simulink model "testEmplanner_cs"  (R2021b)
settings: Solver=ode5  StartTime=0.0  StopTime=60  FixedStep=1/1000  RelTol=1e-3
PreLoadFcn:
  | mbxruntime.callbacks.PreLoadFcn(bdroot);
PostLoadFcn:
  | mbxruntime.callbacks.PostLoadFcn(bdroot);
InitFcn:
  | mbxruntime.callbacks.InitFcn(bdroot);
StartFcn:
  | mbxruntime.callbacks.StartFcn(bdroot);
StopFcn:
  | mbxruntime.callbacks.StopFcn(bdroot);
model workspace (MAT data in the model file):
  mbox_table : object (value not decoded)
  model_closed = 0
  sim_status = 0
values from neighbouring files (symbols this model uses):
  c_factor = 43.75    [emplanner_init.m]
  cf = -175016    [emplanner_init.m]
  cr = -130634    [emplanner_init.m]
  global_path_x = [-1.1448 -0.145417744933 0.852705365581 1.84955224935 2.84511712279 3.83939835808 4.83239585569 5.82411007764 6.81454169183 7.80369144113 8.79156009523 9.77814843293 ... (3001 elements, 3001x1)]    [global_path.mat]
  global_path_y = [14.6488 14.6488 14.6488 14.6488 14.6488 14.6488 14.6488 14.6488 14.6488 14.6488 14.6488 14.6488 ... (3001 elements, 3001x1)]    [global_path.mat]
  KD_PID_distance = 0.0    (= 0)    [emplanner_init.m]
  KD_PID_speed = 0    [emplanner_init.m]
  KI_PID_distance = 0.0    (= 0)    [emplanner_init.m]
  KI_PID_speed = 0    [emplanner_init.m]
  KP_PID_distance = 0.5    [emplanner_init.m]
  KP_PID_speed = 1.8    [emplanner_init.m]
  la = 1.265    [emplanner_init.m]
  lb = 2.947-1.265    (= 1.682)    [emplanner_init.m]
  LQR_K1 = k(:,1)'    [emplanner_init.m]
  LQR_K2 = k(:,2)'    [emplanner_init.m]
  LQR_K3 = k(:,3)'    [emplanner_init.m]
  LQR_K4 = k(:,4)'    [emplanner_init.m]
  m = 2020    [emplanner_init.m]
  rack_displacement = [-39.14 , -37.2 , -35.29 , -33.43 , -31.6 , -29.81 , -28.06 , -26.34 , -24.66 ,      -23.01 , -21.38 , -19.79 , -18.23 , -16.69 , -15.18 , -13.7 , -12.23 , -10.8 , -9.38 , -7.98 ,     -6.61 , -5.25 , -3.91 , -2.59 , -1.29 , 0 , 1.27 , 2.54 , 3.78 , 5.02 , 6.24 , 7.46 , 8.66 ,      9.86 , 11.05 , 12.24 , 13.41 , 14.59 , 15.76 , 16.92 , 18.09 , 19.25 , 20.42 , 21.59 , 22.76 ,      23.93 , 25.11 , 26 ...(+26 chars)    [emplanner_init.m]
  right_wheel_ground = [-70 ,-67.2 , -64.4 , -61.6 , -58.8 , -56 , -53.2 , -50.4 , -47.6 , -44.8 , -42 ,      -39.2 , -36.4 , -33.6 , -30.8 , -28 , -25.2 , -22.4 , -19.6 , -16.8 , -14 , -11.2 , -8.4 , -5.6 ,      -2.8 , 0 , 2.8 , 5.6 , 8.4 , 11.2 , 14 , 16.8 , 19.6 , 22.4 , 25.2 , 28 , 30.8 , 33.6 , 36.4 ,      39.2 , 42 , 44.8 , 47.6 , 50.4 , 53.2 , 56 , 58.8 , 61.6 , 64.4 , 67.2 , 70 ]    [emplanner_init.m]
  vx_break_point = zeros(1,5000)    [emplanner_init.m]
undefined symbols (not defined in the file or in its folder): aubr, DiscIntNeverNeededParam, tablebr, vubr, warningInitialVelocity, x0
libraries: simulink x19, PreScanSimulinkLibrary x17, simulink_extras x6, Solver_SF x1
(part 12 of 14)

== matlab function testEmplanner_cs/Audi_A8_Sedan_1/decision&planning module/referenceline provider/MATLAB Function5 ==
  data: x_set input; match_point_index_set output; y_set input; frenet_path_x input; frenet_path_y input; frenet_path_heading input; frenet_path_kappa input; proj_x_set output; proj_y_set output; proj_heading_set output; proj_kappa_set output
function [match_point_index_set,proj_x_set,proj_y_set,proj_heading_set,proj_kappa_set] = ...
	fcn(x_set,y_set,frenet_path_x,frenet_path_y,frenet_path_heading,frenet_path_kappa)
	
%该函数将批量计算x_set,y_set中(x,y) 在frenet坐标系下的投影信息
%输入： x_set，y_set 待投影的点的集合
	%x_set,y_set,frenet_path_x,frenet_path_y,frenet_path_heading,frenet_path_kappa
	%曲线在直角坐标系下的x,y,heading,kappa
%输出：math_point_index_set 匹配点在frenet_path下的编号的集合（即从全局路径的第一个点开始数，第几个点是匹配点）

%由于事先不知道x_set中有多少个点需要投影，因此事先声明一个最大数量的点作为缓冲

n = 128;
%并且不知道投影点的数量，所以也不知道输出的数量，因此输出也要做缓冲，用nan表示不存在的点
%初始化输出最多为128个点。
%输出初始化
match_point_index_set = ones(n,1) * nan;
proj_x_set = ones(n,1) * nan;
proj_y_set = ones(n,1) * nan;
proj_heading_set = ones(n,1) * nan;
proj_kappa_set = ones(n,1) * nan;

%找匹配点，需要利用上一个周期的结果作为下一个周期遍历的起点，因此需要声明两个全局变量
persistent is_first_run;
persistent pre_match_point_index_set;%bug :pre_match_point_index(i) 未必代表的是第i个障碍物的match_point_index
persistent pre_frenet_path_x;
persistent pre_frenet_path_y;
persistent pre_frenet_path_heading;
persistent pre_frenet_path_kappa;
persistent pre_x_set;
persistent pre_y_set;
%算法主函数入口

if isempty(is_first_run)
	% 该if分支表示函数首次运行
	is_first_run = 0; %赋值
	pre_frenet_path_x = frenet_path_x;
	pre_frenet_path_y = frenet_path_y;
	pre_frenet_path_heading = frenet_path_heading;
	pre_frenet_path_kappa = frenet_path_kappa;
	%记录首次运行计算的匹配点的结果供下个周期运行，先初始化
	pre_match_point_index_set = ones(n,1) * nan;
	
	%对x_set,y_set的点做遍历，找到他们的匹配点
	for i = 1 : length(x_set)
        if isnan(x_set(i))
            break;
        end
	%首次运行时，没有任何提示，只能从frenet_path的第一个点开始找
	start_search_index = 1;
	%声明increa_count,用于表示在遍历时distance连续增大的次数
	increase_count = 0;
	%开始遍历
	min_distance = inf;
	for j = start_search_index : length(frenet_path_x)
		distance = (x_set(i) - frenet_path_x(j))^2 + (y_set(i) - frenet_path_y(j))^2;
		%处理最小值
		if distance < min_distance
			min_distance = distance;
			match_point_index_set(i) = j; %math_point_index_set存放匹配点的序号
			increase_count = 0;
		else
			increase_count = increase_count + 1;
		end
		% 如果连续distanc增加50次,就不要再遍历了，节省时间
		if increase_count > 50 
			break;
		end	
	end
	%如何通过匹配点计算投影点，参考《自动驾驾驶控制算法第七讲》
	%或者《自动驾驶决策规划算法》第一章第三节
		
	%取出匹配点的编号
	match_point_index = match_point_index_set(i);
		
	%取出匹配点信息
	match_point_x = frenet_path_x(match_point_index);
	match_point_y = frenet_path_y(match_point_index);
	match_point_heading = frenet_path_heading(match_point_index);
	match_point_kappa = frenet_path_kappa(match_point_index);
		
	% 计算匹配点的位置向量和方向向量
	vector_match_point = [match_point_x;match_point_y];%位置向量
	vector_match_point_direction = [cos(match_point_heading);sin(match_point_heading)];%方向向量，全局坐标系下（大地坐标系）
		
	%声明待投影点的位矢
	vector_r = [x_set(i);y_set(i)];
		
	%通过匹配点计算投影点
	vector_d = vector_r - vector_match_point;
	ds = vector_d' * vector_match_point_direction;
	vector_proj_point = vector_match_point + ds * vector_match_point_direction;
	proj_heading = match_point_heading + match_point_kappa * ds;
	proj_kappa = match_point_kappa;
		
	%计算结果输出 
	proj_x_set(i) = vector_proj_point(1);
	proj_y_set(i) = vector_proj_point(2);
	proj_heading_set(i) = proj_heading;
	proj_kappa_set(i) = proj_kappa;
   end
	
	%匹配点的计算结果保存，供下一个周期使用
	pre_match_point_index_set = match_point_index_set;
	pre_x_set = x_set;
	pre_y_set = y_set;
else
	% 此分支不是首次运行
	
	%对每个x_set上的点做处理
	for i = 1 : length(x_set)
		%不是首次运行，对于点x_set(i),y_set(i)来说，
		%start_search_index = pre_match_point_index_set(i)
		start_search_index = pre_match_point_index_set(i);%上个周期匹配点的编号作为本周期搜索的起点
		%判断帧与帧之间的障碍物是否为同一个
		square_dis = (x_set(i) - pre_x_set(i))^2 + (y_set(i) - pre_y_set(i))^2;
		if square_dis > 36	 
			% 帧与帧之间的物体位置距离过大，认为是两个障碍物
			start_search_index = nan;
		end
        %
        % 对于障碍物的检测而言，当感知第一次检测到障碍物时，算法并不是首次运行，此时
        % pre_match_point_set的值是nan，如果还用上一个时刻的结果作为本周期搜索的起点
        % 必然会出问题，所以要修改
        % 声明 increase_count_limit
        increase_count_limit = 5;
        if isnan(start_search_index)
	        % 没有上个周期的结果，那么就不能只检查5次
	        increase_count_limit = 50;
	        % 搜索的起点也要设为 1
	        start_search_index = 1;
        end
		%声明increa_count,用于表示在遍历时distance连续增大的次数
		increase_count = 0;
		%开始遍历
		
		%这里多了一个步骤，判断遍历的方向
		%计算上个周期匹配点的位失
		vector_pre_match_point = [pre_frenet_path_x(start_search_index); pre_frenet_path_y(start_search_index)];
		vector_pre_match_point_direction = ...
			[cos(pre_frenet_path_heading(start_search_index));sin(pre_frenet_path_heading(start_search_index))];
		
		% 判断遍历的方向
		flag = ([x_set(i);y_set(i)] - vector_pre_match_point)' * vector_pre_match_point_direction;
		
		min_distance = inf;
		
		if flag > 0.001 
			for j = start_search_index : length(frenet_path_x)
				distance = (x_set(i) - frenet_path_x(j))^2 + (y_set(i) - frenet_path_y(j))^2;
				%处理最小值
				if distance < min_distance
					min_distance = distance;
					match_point_index_set(i) = j; %math_point_index_set存放匹配点的序号
					increase_count = 0;
				else
					increase_count = increase_count + 1;
				end
				% 如果连续distanc增加increase_count_limit次,就不要再遍历了，节省时间
				if increase_count > increase_count_limit
					break;
				end
			end
		elseif flag < -0.001
			for j = start_search_index :-1: 1
				distance = (x_set(i) - frenet_path_x(j))^2 + (y_set(i) - frenet_path_y(j))^2;
				%处理最小值
				if distance < min_distance
					min_distance = distance;
					match_point_index_set(i) = j; %math_point_index_set存放匹配点的序号
					increase_count = 0;
				else
					increase_count = increase_count + 1;
				end
				% 如果连续distanc增加50次,就不要再遍历了，节省时间
				if increase_count > increase_count_limit 
					break;
				end
			end
		else
			match_point_index_set(i) = start_search_index;
		end
			
		%如何通过匹配点计算投影点，参考《自动驾驾驶控制算法第七讲》
		%或者《自动驾驶决策规划算法》第一章第三节
		
		%取出匹配点的编号
		match_point_index = match_point_index_set(i);
		
		%取出匹配点信息
		match_point_x = frenet_path_x(match_point_index);
		match_point_y = frenet_path_y(match_point_index);
		match_point_heading = frenet_path_heading(match_point_index);
		match_point_kappa = frenet_path_kappa(match_point_index);
		
		% 计算匹配点的位置向量和方向向量
		vector_match_point = [match_point_x;match_point_y];%位置向量
		vector_match_point_direction = [cos(match_point_heading);sin(match_point_heading)];%方向向量
		
		%声明待投影点的位矢
		vector_r = [x_set(i);y_set(i)];
		
		%通过匹配点计算投影点
		vector_d = vector_r - vector_match_point;
		ds = vector_d' * vector_match_point_direction;
		vector_proj_point = vector_match_point + ds * vector_match_point_direction;
		proj_heading = match_point_heading + match_point_kappa * ds;
		proj_kappa = match_point_kappa;
		
		%计算结果输出 
		proj_x_set(i) = vector_proj_point(1);
		proj_y_set(i) = vector_proj_point(2);
		proj_heading_set(i) = proj_heading;
		proj_kappa_set(i) = proj_kappa;
	end
	
	%匹配点的计算结果保存，供下一个周期使用
	pre_match_point_index_set = match_point_index_set;
	pre_frenet_path_x = frenet_path_x;
	pre_frenet_path_y = frenet_path_y;
	pre_frenet_path_heading = frenet_path_heading;
	pre_frenet_path_kappa = frenet_path_kappa;
	pre_x_set = x_set;
	pre_y_set = y_set;
end

== matlab function testEmplanner_cs/Audi_A8_Sedan_1/decision&planning module/EM Planner/path planning task/path planning with quadratic programming (qp) ==
  data: qp_path_s output; l_min input; qp_path_l output; l_max input; w_cost_l input; w_cost_dl input; w_cost_ddl input; w_cost_dddl input; qp_path_dl output; w_cost_centre input; w_cost_end_l input; w_cost_end_dl input; w_cost_end_ddl input; host_d1 input; host_d2 input; host_w input; plan_start_s input; plan_start_l input; plan_start_dl input; plan_start_ddl input; qp_path_ddl output; delta_dl_max input; delta_ddl_max input
function [qp_path_s,qp_path_l,qp_path_dl,qp_path_ddl] = ...
	fcn(l_min,l_max,w_cost_l,w_cost_dl,w_cost_ddl,w_cost_dddl,w_cost_centre,w_cost_end_l,w_cost_end_dl,w_cost_end_ddl,...
		host_d1,host_d2,host_w,...
		plan_start_s,plan_start_l,plan_start_dl,plan_start_ddl,...
		delta_dl_max,delta_ddl_max)
	%路径规划算法：二次规划算法
	% 0.5 * x‘Hx + f'* x = min
	% subject to : A*x <= b
	%  			   Aeq*x = beq
	% 			   lb <= x <= ub
	%输入：l_min,l_max 点的凸空间
	% 	  w_cost_l 参考点代价
	% 	  w_cost_dl ddl dddl 光滑性代价
	%	  w_cost_centre 凸空间中央代价
	% 	  w_cost_end_l dl ddl 终点的状态代价(希望path的终点状态为0，0，0)
	% 	  host_d1,host_d2,host_w 质心到前轴的距离，质心到后轴的距离，车辆的宽度
	%	  plan_start_l,plan_start_dl,plan_start_ddl 规划起点的l,dl,ddl
	%
	%输出 qp_path_s,qp_path_l，qp_path_dl,qp_path_ddl 二次规划输出的曲线
	coder.extrinsic("quadprog");

	%待优化变量的数量
	n = 20;

	%输出初始化
	qp_path_l = zeros(n,1);
	qp_path_dl = zeros(n,1);
	qp_path_ddl = zeros(n,1); 
	qp_path_s = zeros(n,1);

	% H_L H_DL H_DDL H_DDDL Aeq beq A b 初始化

	H_L = zeros(3*n,3*n);
	H_DL = zeros(3*n,3*n);
	H_DDL = zeros(3*n,3*n);
	H_DDDL = zeros(n-1,3*n);
	H_CENTRE = zeros(3*n,3*n);
	H_L_END = zeros(3*n,3*n);
	H_DL_END = zeros(3*n,3*n);
	H_DDL_END = zeros(3*n,3*n);
	Aeq = zeros(2*n-2,3*n);
	beq = zeros(2*n-2,1);
	A = zeros(8*n,3*n);
	b = zeros(8*n,1);
	%更新加入 dl(i+1) - dl(i) ddl(i+1) - ddl(i)的约束
	A_dl_minus = zeros(n - 1,3*n);
	b_dl_minus = zeros(n - 1,1);
	A_ddl_minus = zeros(n - 1,3*n);
	b_ddl_minus = zeros(n - 1,1);
	for i = 1:n-1
	    row = i;
	    col = 3*i - 2;
	    A_dl_minus(row,col:col+5) = [0 -1 0 0 1 0];
	    b_dl_minus(row) = delta_dl_max;
	    A_ddl_minus(row,col:col+5) = [0 0 -1 0 0 1];
	    b_ddl_minus(row) = delta_ddl_max;
	end
	% -max < a*x < max => ax < max && -ax < -(-max)
	A_minus = [A_dl_minus;
	          -A_dl_minus;
	           A_ddl_minus;
	          -A_ddl_minus];
	b_minus = [b_dl_minus;
	           b_dl_minus;
	          b_ddl_minus;
	          b_ddl_minus]; 

	%  期望的终点状态
	end_l_desire = 0;
	end_dl_desire = 0;
	end_ddl_desire = 0;

	%Aeq_sub 
	ds = 3;%纵向间隔
	for i = 1:n
		qp_path_s(i) = plan_start_s + (i-1)*ds;
	end

	Aeq_sub = [1 ds ds^2/3 -1 0 ds^2/6;
	           0 1  ds/2   0 -1 ds/2];
	% A_sub;
	d1 = host_d1;
	d2 = host_d2;
	w = host_w;
	A_sub = [1  d1 0;
	         1  d1 0;
	         1 -d2 0;
	         1 -d2 0;
	        -1 -d1 0;
	        -1 -d1 0;
	        -1  d2 0;
	        -1  d2 0];
	% 生成Aeq
	for i = 1:n-1
		%计算分块矩阵左上角的行和列
		row = 2 * i -1;
		col = 3 * i -2;
		Aeq(row:row+1,col:col+5) = Aeq_sub;
	end

	%生成A
	for i = 2 : n
		%计算生成A_sub
		row = 8 * i - 7;
		col = 3 * i - 2;
		A(row:row + 7,col:col + 2) = A_sub;
	end

	%生成b
	%视频里用的找到（s(i)- d2,s(i) + d1)的方法过于保守，在这里舍弃掉
	%只要找到四个角点对应的l_min,l_max即可

	front_index = ceil(d1 / ds);
	back_index = ceil(d2 / ds); %ceil 向上取整，ceil(3) = 3 , ceil (3.1) = 4;
	%生成b
	for i = 2 : n 
		% 左前 右前的index = min(i + front_index,60);
		% 左后 右后的index = max(i - back_index,1);
	 	% l_min l_max 都是60个点
		index1 = min(3 * i - 2 + front_index,n);
		index2 = max(3 * i - 2 - back_index,1);
		b(8 * i - 7:8 * i,1) = [l_max(index1) - w/2;
								l_max(index1) + w/2;
								l_max(index2) - w/2;
								l_max(index2) + w/2;
								-l_min(index1) + w/2;
								-l_min(index1) - w/2;
								-l_min(index2) + w/2;
								-l_min(index2) - w/2;];
	end
	%生成 lb ub主要对规划的起点做约束
	lb = ones(3 * n ,1) * -inf;
	ub = ones(3 * n, 1) * inf;
	lb(1) = plan_start_l;
	lb(2) = plan_start_dl;
	lb(3) = plan_start_ddl;
	ub(1) = lb(1);
	ub(2) = lb(2);
	ub(3) = lb(3);
	for i = 2:n
	    lb(3*i - 1) = - 2; %约束 l'
	    ub(3*i - 1) = 2;
	    lb(3*i) = -0.1; %约束 l''
	    ub(3*i) = 0.1;
	end
	%生成H_L H_DL H_DDL H_CENTRE
	for i = 1 : n
		H_L(3 * i - 2,3 * i -2) = 1;
		H_DL(3 * i - 1,3 * i -1) = 1;
		H_DDL(3 * i,3 * i) = 1;
	end
	H_CENTRE = H_L;

	%生成H_DDDL；
	H_dddl_sub = [0 0 1 0 0 -1];
	for i = 1 : n - 1
		row = i;
		col = 3 * i - 2;
		H_DDDL(row,col:col+5) = H_dddl_sub;
	end

	%生成H_L_END H_DL_END H_DDL_END
	H_L_END(3 * n -2,3 * n - 2) = 1;
	H_DL_END(3 * n - 1,3 * n -1) = 1;
	H_DDL_END(3 * n,3 * n) = 1;

	%生成二次规划的H 因为ds != 1 所以dddl = delta_ddl/ds

	H = w_cost_l * (H_L' * H_L) + w_cost_dl * (H_DL' * H_DL) + w_cost_ddl * (H_DDL' * H_DDL) ...
		+ w_cost_dddl * (H_DDDL' * H_DDDL) /ds + w_cost_centre * (H_CENTRE' * H_CENTRE) + w_cost_end_l * (H_L_END' * H_L_END) ...
		+ w_cost_end_dl * (H_DL_END' * H_DL_END) + w_cost_ddl * (H_DDL_END' * H_DDL_END);

	H = 2 * H;
	%生成 f
	f = zeros(3 * n,1);
	centre_line = 0.5 * (l_min + l_max);
	% 尽可能靠近centre_line,  (x-centre)^2 = x^2 - 2 * x * centre + centre^2
	for i = 1 : n
		f(3 * i - 2) = -2 * centre_line(3 * i -2);
	end
	% 避免centreline权重过大影响轨迹平顺性
	for i = 1:n
	    if abs(f(i)) > 0.3
	        f(i) = w_cost_centre * f(i);
	    end
	end
	% 终点要接近end_l dl ddl desire
	f(3*n - 2) = f(3*n - 2) -2 * end_l_desire * w_cost_end_l;
	f(3*n - 1) = f(3*n - 1) -2 * end_dl_desire * w_cost_end_dl;
	f(3*n) = f(3*n) -2 * end_ddl_desire * w_cost_end_ddl;

	X = quadprog(H,f,[A;A_minus],[b;b_minus],Aeq,beq,lb,ub);
	%这里并不好，没有对曲率做强制约束
	%可以用|dl(i+1) - dl(i)| / ds <= kappa_max 近似做曲率约束，因为精确曲率约束是非线性约束

	for i = 1:n
	    qp_path_l(i) = X(3*i - 2);
	    qp_path_dl(i) = X(3*i - 1);
	    qp_path_ddl(i) = X(3*i);
	end

end

== matlab function testEmplanner_cs/Audi_A8_Sedan_1/decision&planning module/EM Planner/path planning task/MATLAB Function1 ==
  data: qp_path_s input; qp_path_s_final output; qp_path_l input; qp_path_dl input; qp_path_ddl input; qp_path_l_final output; qp_path_dl_final output; qp_path_ddl_final output
function [qp_path_s_final,qp_path_l_final,qp_path_dl_final,qp_path_ddl_final] = fcn(qp_path_s,qp_path_l,qp_path_dl,qp_path_ddl)
%该函数将增密qp_path
n_init = 20;
%增密点的个数
n = 501;
%输出初始化
qp_path_s_final = zeros(n,1);
qp_path_l_final = zeros(n,1);
qp_path_dl_final = zeros(n,1);
qp_path_ddl_final = zeros(n,1);
ds = (qp_path_s(end) - qp_path_s(1)) / (n - 1);
index = 1;
for i = 1 : n
	x = qp_path_s(1) + (i - 1) * ds;
	qp_path_s_final(i) = x;
	while x >= qp_path_s(index) 
		index = index + 1 ;
		if index == n_init
			break;
		end
	end
	% while循环退出条件是 x < qp_path_s(index) ,所以x对应的前一个s的编号是 index-1  后一个是index
	pre = index - 1;
	cur = index;
	% 计算前一个点的 l l' l'' ds和后一个点的l''
	delta_s = x - qp_path_s(pre);
	l_pre = qp_path_l(pre);
	dl_pre = qp_path_dl(pre);
	ddl_pre = qp_path_ddl(pre);
	ddl_cur = qp_path_ddl(cur);
	%分段加速度优化算法
	% li+1 = li + li' * ds + 0.5 * li'' * ds^2 + 1/6 * (li+1'' - li'')*ds^2;
	% li+1' = li' + li'' * ds + 0.5 * (li+1'' - li'') * ds;
	qp_path_l_final(i) = l_pre + dl_pre * delta_s + (1/3) * ddl_pre * delta_s^2 + (1/6) * ddl_cur * delta_s^2;
	qp_path_dl_final(i) = dl_pre + 0.5 * ddl_pre * delta_s + 0.5 * ddl_cur * delta_s;
	qp_path_ddl_final(i) = ddl_pre + (ddl_cur - ddl_pre) * delta_s / (qp_path_s(cur) - qp_path_s(pre)); %%线性插值
	%  因为此时x的后一个编号是index 必有x < qp_path_s(index)，在下一个循环中 x = x + ds 也必大于
	%  qp_path_s(index),这样就进不了while循环，所以index要回退一位
	index = index - 1;
end

== matlab function testEmplanner_cs/Audi_A8_Sedan_1/decision&planning module/EM Planner/MATLAB Function ==
  data: trajectory_heading_final input; y output
function y = fcn(trajectory_heading_final)
y = zeros(421,1);
y(1) = trajectory_heading_final(1);
for i = 2:421
    y(i) = y(i-1) + sin(trajectory_heading_final(i) - trajectory_heading_final(i-1));
end

== matlab function testEmplanner_cs/Audi_A8_Sedan_1/control module/control main/lateral control LQR/err_kappa_calculate_module ==
  data: x input; y input; phi input; vx input; vy input; phi_dot input; xr input; yr input; thetar input; kappar input; err output; es output; s_dot output
function [err,es,s_dot] = fcn(x,y,phi,vx,vy,phi_dot,xr,yr,thetar,kappar)
    
    tor=[cos(thetar);sin(thetar)];
    nor=[-sin(thetar);cos(thetar)];
    d_err=[x-xr;y-yr];
    ed=nor'*d_err;
    es=tor'*d_err;
    %projection_point_thetar=thetar(dmin);%apollo
    projection_point_thetar=thetar+kappar*es;
    ed_dot=vy*cos(phi-projection_point_thetar)+vx*sin(phi-projection_point_thetar);
    %%%%%%%%%
    ephi=sin(phi-projection_point_thetar);
    %%%%%%%%%
    ss_dot=vx*cos(phi-projection_point_thetar)-vy*sin(phi-projection_point_thetar);
    s_dot=ss_dot/(1-kappar*ed);
    ephi_dot=phi_dot-kappar*s_dot;
    err=[ed;ed_dot;ephi;ephi_dot];
    
    
    
    
    
    
    
    
    
    
    
    


end

== matlab function testEmplanner_cs/Audi_A8_Sedan_1/control module/control main/lateral control LQR/feed_forword_control ==
  data: vx input; a input; forword_angle output; b input; m input; cf input; cr input; k input; kr input
function forword_angle = fcn(vx,a,b,m,cf,cr,k,kr)
    forword_angle=kr*(a+b-b*k(3)-(m*vx*vx/(a+b))*((b/cf)+(a/cr)*k(3)-(a/cr)));
end

== matlab function testEmplanner_cs/Audi_A8_Sedan_1/control module/control main/chassic steering system/MATLAB Function ==
  data: u input; right_steer output; la input; lb input
function right_steer = fcn(u,la,lb)
if abs(u)<1e-2
   right_steer = u;
else
   R =  (la+lb)/tan(u);
   right_steer = atan((la+lb)/(R+1.624/2));
end

== matlab function testEmplanner_cs/Audi_A8_Sedan_1/control module/control main/lateral control LQR/feedback_control+feedforword_control ==
  data: k input; angle output; err input; forword_angle input
function angle = fcn(k,err,forword_angle)

    angle=-k*err+forword_angle;
end

== matlab function testEmplanner_cs/Audi_A8_Sedan_1/control module/control main/lateral control LQR/calc lqr K ==
  data: k1 input; k output; k2 input; k3 input; k4 input; vx input
function k = fcn(k1,k2,k3,k4,vx)
    if abs(vx) < 0.1 
        k = [0,0,0,0];
    else
        k =[k1,k2,k3,k4];
    end

== matlab function testEmplanner_cs/Audi_A8_Sedan_1/control module/control main/lateral control LQR/predict_module ==
  data: x input; pred_x_ctrl output; y input; phi input; vx input; vy input; phi_dot input; ts input; pred_y_ctrl output; pred_yaw_ctrl output; pred_vx_ctrl output; pred_vy_ctrl output; pred_yaw_dot_ctrl output
function [pred_x_ctrl,pred_y_ctrl,pred_yaw_ctrl,pred_vx_ctrl,pred_vy_ctrl,pred_yaw_dot_ctrl] = fcn(x,y,phi,vx,vy,phi_dot,ts)
    pred_x_ctrl=x+vx*ts*cos(phi)-vy*ts*sin(phi);
    pred_y_ctrl=y+vy*ts*cos(phi)+vx*ts*sin(phi);
    pred_yaw_ctrl=phi;
    pred_vx_ctrl=vx;
    pred_vy_ctrl=vy;
    pred_yaw_dot_ctrl=phi_dot;
end

== matlab function testEmplanner_cs/Audi_A8_Sedan_1/decision&planning module/EM Planner2/Cartesian2Frenet/MATLAB Function ==
  data: x_set input; s_set output; y_set input; frenet_path_x input; frenet_path_y input; proj_x_set input; proj_y_set input; proj_heading_set input; proj_match_point_index_set input; index2s input; l_set output
function [s_set,l_set] = fcn(x_set,y_set,frenet_path_x,frenet_path_y,...
    proj_x_set,proj_y_set,proj_heading_set,proj_match_point_index_set,index2s)
    %该函数将计算世界坐标系下的x_set，y_set上的点在frenet_path下的坐标s l
    %输入 x_set,y_set 待坐标转换的点
    %     frenet_path_x,frenet_path_y   frenet坐标轴
    %     proj_x,y,heading,kappa,proj_match_point_index 待坐标转换的点的投影点的信息
    %     index2s   frenet_path的index与s的转换表

    % 由于不知道有多少个点需要做坐标转换，所以需要做缓冲
    n = 128;%最多处理128个点
    %输出初始化
    s_set = ones(n,1)*nan;
    l_set = ones(n,1)*nan;
    for i = 1:length(x_set)
        if isnan(x_set(i))
            break;
        end
        %计算s，写个子函数
        s_set(i) = CalcSFromIndex2S(index2s,frenet_path_x,frenet_path_y,proj_x_set(i),proj_y_set(i),...
            proj_match_point_index_set(i));
        n_r = [-sin(proj_heading_set(i));cos(proj_heading_set(i))];
        r_h = [x_set(i);y_set(i)];
        r_r = [proj_x_set(i);proj_y_set(i)];
        l_set(i) = (r_h - r_r)'*n_r;
    end
end

function s = CalcSFromIndex2S(index2s,path_x,path_y,proj_x,proj_y,proj_match_point_index)
  %该函数将计算当指定index2s的映射关系后，计算点proj_x,proj_y的弧长
  vector_1 = [proj_x;proj_y] - [path_x(proj_match_point_index);path_y(proj_match_point_index)];
  %这里要考虑的更全面一些，因为要考虑到proj_match_point_index有可能在path的起点或终点
  if (proj_match_point_index < length(path_x))
      vector_2 = [path_x(proj_match_point_index + 1);path_y(proj_match_point_index + 1)] - ...
          [path_x(proj_match_point_index);path_y(proj_match_point_index)];
  else
      vector_2 = [path_x(proj_match_point_index);path_y(proj_match_point_index)] - ...
          [path_x(proj_match_point_index - 1);path_y(proj_match_point_index - 1)];
  end
  
  if vector_1'*vector_2 > 0
      s = index2s(proj_match_point_index) + sqrt(vector_1'*vector_1);
  else
      s = index2s(proj_match_point_index) - sqrt(vector_1'*vector_1);
  end
  
  
end

== matlab function testEmplanner_cs/Audi_A8_Sedan_1/decision&planning module/EM Planner2/Cartesian2Frenet/MATLAB Function1 ==
  data: l_set input; s_dot_set output; vx_set input; vy_set input; proj_heading_set input; proj_kappa_set input; l_dot_set output; dl_set output
function [s_dot_set,l_dot_set,dl_set] = fcn(l_set,vx_set,vy_set,proj_heading_set,proj_kappa_set)
%该函数将计算frenet坐标系下的s_dot, l_dot, dl/ds
n = 128;
% 输出初始化
s_dot_set = ones(n,1)*nan;
l_dot_set = ones(n,1)*nan;
dl_set = ones(n,1)*nan;

for i = 1 : length(l_set)
    if isnan(l_set(i))
        break;
    end
    v_h = [vx_set(i);vy_set(i)];
    n_r = [-sin(proj_heading_set(i));cos(proj_heading_set(i))];
    t_r = [cos(proj_heading_set(i));sin(proj_heading_set(i))];
    l_dot_set(i) = v_h'*n_r;
    s_dot_set(i) = v_h'*t_r/(1 - proj_kappa_set(i)*l_set(i));
    %%%向量法做cartesian与frenet的转换要更简单，但是也有缺点，向量法必须依赖速度加速度
    %l' = l_dot/s_dot 但是如果s_dot = 0 此方法就失效了
    if abs(s_dot_set(i)) < 1e-6
        dl_set(i) = 0;
    else
        dl_set(i) = l_dot_set(i)/s_dot_set(i);
    end
end

== matlab function testEmplanner_cs/Audi_A8_Sedan_1/decision&planning module/EM Planner2/Cartesian2Frenet/MATLAB Function2 ==
  data: ax_set input; s_dot2_set output; ay_set input; proj_heading_set input; proj_kappa_set input; l_set input; s_dot_set input; dl_set input; l_dot2_set output; ddl_set output
function [s_dot2_set,l_dot2_set,ddl_set] = fcn(ax_set,ay_set,proj_heading_set,proj_kappa_set,l_set,s_dot_set,dl_set)
%由于不知道有多少个点需要做坐标转换，设一个最大值做缓冲
n = 128;
% 输出初始化
s_dot2_set = ones(n,1)*nan;
l_dot2_set = ones(n,1)*nan;
ddl_set = ones(n,1)*nan;

for i = 1:length(l_set)
    if isnan(l_set(i))
       break;
    end
    a_h = [ax_set(i);ay_set(i)];
    n_r = [-sin(proj_heading_set(i));cos(proj_heading_set(i))];
    t_r = [cos(proj_heading_set(i));sin(proj_heading_set(i))];
    %近似认为dkr/ds 为0 简化计算
    l_dot2_set(i) = a_h'*n_r - proj_kappa_set(i) * (1 - proj_kappa_set(i) * l_set(i)) * s_dot_set(i)^2;
    s_dot2_set(i) = (1/(1 - proj_kappa_set(i) * l_set(i)))* (a_h' * t_r + 2 * proj_kappa_set(i) * dl_set(i) * s_dot_set(i)^2);
    % 要考虑加速度为0的情况
    if (s_dot2_set(i) < 1e-6)
        ddl_set(i) = 0;
    else
        ddl_set(i) = (l_dot2_set(i) - dl_set(i)*s_dot2_set(i))/(s_dot_set(i)^2);
    end
end

== matlab function testEmplanner_cs/Audi_A8_Sedan_1/decision&planning module/EM Planner2/MATLAB Function1 ==
  data: x_set input; match_point_index_set output; y_set input; frenet_path_x input; frenet_path_y input; frenet_path_heading input; frenet_path_kappa input; proj_x_set output; proj_y_set output; proj_heading_set output; proj_kappa_set output
function [match_point_index_set,proj_x_set, proj_y_set,proj_heading_set,proj_kappa_set] = ...
    fcn(x_set,y_set,frenet_path_x,frenet_path_y,frenet_path_heading,frenet_path_kappa)
%该函数将批量计算x_set，y_set中的xy，在frenet_path下的投影的信息
%输入 x_set,y_set，待投影的点的集合
%x_set,y_set,frenet_path_x,frenet_path_y,frenet_path_heading,frenet_path_kappa
%曲线在直角坐标系下的x，y，heading，kappa
%输出：match_point_index_set 匹配点在frenet_path下的编号的集合(即从全局路径第一个点开始数，第几个点是匹配点)
%     proj_x y heading kappa 投影的x,y,heading,kappa的集合

% 由于事先不知道x_set中到底有多少个点需要投影，因此事先声明一个最大的数量的点作为缓冲
n = 128;
% 并且由于不知道投影点的个数，所以也不知道输出的个数，因此输出也要做缓冲，用nan表示不存在的点
% 输出最多输出128个
% 输出初始化
match_point_index_set = ones(n,1) * nan;
proj_x_set = ones(n,1) * nan;
proj_y_set = ones(n,1) * nan;
proj_heading_set = ones(n,1) * nan;
proj_kappa_set = ones(n,1) * nan;

%找匹配点，需要利用上一个周期的结果作为下一个周期遍历的起点，因此需要声明两个全局变量
persistent is_first_run;
persistent pre_match_point_index_set;
persistent pre_frenet_path_x;
persistent pre_frenet_path_y;
persistent pre_frenet_path_heading;
persistent pre_frenet_path_kappa;
%算法主函数入口

if isempty(is_first_run)
    %该if分支表示函数首次运行
    is_first_run = 0;
    pre_frenet_path_x = frenet_path_x;
    pre_frenet_path_y = frenet_path_y;
    pre_frenet_path_heading = frenet_path_heading;
    pre_frenet_path_kappa = frenet_path_kappa;
    %要记录首次运行计算的匹配点的结果供下个周期运行，先初始化
    pre_match_point_index_set = ones(n,1) * nan;
    %对x_set,y_set的点做遍历，找到他们的匹配点
    for i = 1 : length(x_set)
        if isnan(x_set(i))
            break;
        end
        %首次运行时，没有任何提示，只能从frenet path的第一个点开始找
        start_search_index = 1;
        % 声明increase_count，用于表示在遍历时distance连续增加的个数
        increase_count = 0;
        % 开始遍历
        min_distance = inf;
        for j = start_search_index : length(frenet_path_x)
            distance = (x_set(i) - frenet_path_x(j))^2 + (y_set(i) - frenet_path_y(j))^2;
            if distance < min_distance
                min_distance = distance;
                match_point_index_set(i) = j;
                increase_count = 0;
            else
                increase_count = increase_count + 1;
            end
            %如果distance连续增加50次就不要再遍历了，节省时间
            if increase_count > 50
                break;
            end
        end
        
        %如何通过匹配点计算投影点，请参见《自动驾驶控制算法第七讲》
        %或《自动驾驶决策规划算法》第一章第三节
        
        %取出匹配点的编号
        match_point_index = match_point_index_set(i);
        %取出匹配点的信息
        match_point_x = frenet_path_x(match_point_index);
        match_point_y = frenet_path_y(match_point_index);
        match_point_heading = frenet_path_heading(match_point_index);
        match_point_kappa = frenet_path_kappa(match_point_index);
        %计算匹配点的方向向量与法向量
        vector_match_point = [match_point_x;match_point_y];
        vector_match_point_direction = [cos(match_point_heading);sin(match_point_heading)];
        %声明待投影点的位矢
        vector_r = [x_set(i);y_set(i)];
        
       %通过匹配点计算投影点
       vector_d = vector_r - vector_match_point;
       ds = vector_d' * vector_match_point_direction;
       vector_proj_point = vector_match_point + ds * vector_match_point_direction;
       proj_heading = match_point_heading + match_point_kappa * ds;
       proj_kappa = match_point_kappa;
       %计算结果输出
       proj_x_set(i) = vector_proj_point(1);
       proj_y_set(i) = vector_proj_point(2);
       proj_heading_set(i) = proj_heading;
       proj_kappa_set(i) = proj_kappa;
    end
    %匹配点的计算结果保存，供下一个周期使用
    pre_match_point_index_set = match_point_index_set;
else
    %此if分支表示不是首次运行
    
    %对每个x_set上的点做处理
    for i = 1 : length(x_set)
        %不是首次运行，对于点x_set(i),y_set(i)来说,start_search_index =
        %pre_match_point_index_set(i)
        start_search_index = pre_match_point_index_set(i);%上个周期匹配点的编号作为本周期搜索的起点
        % 声明increase_count，用于表示在遍历时distance连续增加的个数
        %%%%%%%%%
        %对于障碍物检测而言，当感知第一次检测到障碍物时，算法并不是首次运行，此时 
        %pre_match_point_index_set的值是nan，如果还用上一时刻的结果作为本周期搜索的起点
        %必然会出问题，所以要修改
        % 声明increase_count_limit
        increase_count_limit = 5;
        if isnan(start_search_index)
            %没有上个周期的结果，那就不能只检查5次了
            increase_count_limit = 50;
            %搜索起点也要设为1
            start_search_index = 1;
        end
        increase_count = 0;
        % 开始遍历
        %这里多一个步骤，判断遍历的方向
        %计算上个周期匹配点的位矢
        vector_pre_match_point = [pre_frenet_path_x(start_search_index);pre_frenet_path_y(start_search_index)];
        vector_pre_match_point_direction = ...
            [cos(pre_frenet_path_heading(start_search_index));sin(pre_frenet_path_heading(start_search_index))];
        %判断遍历的方向
        flag = ([x_set(i);y_set(i)] - vector_pre_match_point)' * vector_pre_match_point_direction;
        min_distance = inf;
        if flag > 0.001
            for j = start_search_index : length(frenet_path_x)
                distance = (x_set(i) - frenet_path_x(j))^2 + (y_set(i) - frenet_path_y(j))^2;
                if distance < min_distance
                    min_distance = distance;
                    match_point_index_set(i) = j;
                    increase_count = 0;
                else
                    increase_count = increase_count + 1;
                end
                %如果distance连续增加increase_count_limit次就不要再遍历了，节省时间
                if increase_count > increase_count_limit
                    break;
                end
            end
        elseif flag < - 0.001
            for j = start_search_index : -1 : 1
                distance = (x_set(i) - frenet_path_x(j))^2 + (y_set(i) - frenet_path_y(j))^2;
                if distance < min_distance
                    min_distance = distance;
                    match_point_index_set(i) = j;
                    increase_count = 0;
                else
                    increase_count = increase_count + 1;
                end
                %如果distance连续增加increase_count_limit次就不要再遍历了，节省时间
                if increase_count > increase_count_limit
                    break;
                end
            end
        else
            match_point_index_set(i) = start_search_index;
        end
        
        %如何通过匹配点计算投影点，请参见《自动驾驶控制算法第七讲》
        %或《自动驾驶决策规划算法》第一章第三节
        
        %取出匹配点的编号
        match_point_index = match_point_index_set(i);
        %取出匹配点的信息
        match_point_x = frenet_path_x(match_point_index);
        match_point_y = frenet_path_y(match_point_index);
        match_point_heading = frenet_path_heading(match_point_index);
        match_point_kappa = frenet_path_kappa(match_point_index);
        %计算匹配点的方向向量与法向量
        vector_match_point = [match_point_x;match_point_y];
        vector_match_point_direction = [cos(match_point_heading);sin(match_point_heading)];
        %声明待投影点的位矢
        vector_r = [x_set(i);y_set(i)];
        
       %通过匹配点计算投影点
       vector_d = vector_r - vector_match_point;
       ds = vector_d' * vector_match_point_direction;
       vector_proj_point = vector_match_point + ds * vector_match_point_direction;
       proj_heading = match_point_heading + match_point_kappa * ds;
       proj_kappa = match_point_kappa;
       %计算结果输出
       proj_x_set(i) = vector_proj_point(1);
       proj_y_set(i) = vector_proj_point(2);
       proj_heading_set(i) = proj_heading;
       proj_kappa_set(i) = proj_kappa;
  
    end
    %匹配点的计算结果保存，供下一个周期使用
    pre_match_point_index_set = match_point_index_set;
    pre_frenet_path_x = frenet_path_x;
    pre_frenet_path_y = frenet_path_y;
    pre_frenet_path_heading = frenet_path_heading;
    pre_frenet_path_kappa = frenet_path_kappa;
end

== stateflow chart testEmplanner_cs/Audi_A8_Sedan_1/Schedule OS ==
  (default) -> (junction 5)
  (junction 5) -> (junction 9) [order 1] : [i>=100]
  (junction 5) -> (junction 10) [order 2] : {i = i+1;}
  (junction 9) -> (junction 12) : {
      | do_planning;
      | i = 1;
      | }
  (junction 12) -> (junction 10)
  (junction 10) -> (junction 15)
  (junction 15) -> (junction 17) [order 1] : [j>=10]
  (junction 15) -> (junction 21) [order 2] : {j = j+1}
  (junction 17) -> (junction 19) : {
      | do_control;
      | j = 1;
      | }
  (junction 19) -> (junction 21)
  (junction 21) -> (junction 24)
  data: i local =1; j local =1
  events: do_planning output FUNCTION_CALL_EVENT; do_control output FUNCTION_CALL_EVENT

== matlab function testEmplanner_cs/Audi_A8_Sedan_1/decision&planning module/EM Planner2/Frenet2Cartesian ==
  data: s_set input; x_set output; l_set input; dl_set input; ddl_set input; frenet_path_x input; frenet_path_y input; frenet_path_heading input; frenet_path_kappa input; index2s input; y_set output; heading_set output; kappa_set output
function [x_set,y_set,heading_set,kappa_set] = ...
    fcn(s_set,l_set,dl_set,ddl_set,frenet_path_x,frenet_path_y,frenet_path_heading,frenet_path_kappa,index2s)
% 通用算法 frenet转frenet
% 由于不知道有多少个(s,l)要转化成直角坐标，因此做缓冲
% 输出初始化
    x_set = ones(128,1) * nan;
    y_set = ones(128,1) * nan;
    heading_set = ones(128,1) * nan;
    kappa_set = ones(128,1) * nan;
    for i = 1:length(s_set)
        if isnan(s_set(i))
            break;
        end
        % 计算(s,l)在frenet坐标轴上的投影
        [proj_x,proj_y,proj_heading,proj_kappa] = CalcProjPoint(s_set(i),frenet_path_x,frenet_path_y,frenet_path_heading,...
    frenet_path_kappa,index2s);
        nor = [-sin(proj_heading);cos(proj_heading)];
        point = [proj_x;proj_y] + l_set(i) * nor;
        x_set(i) = point(1);
        y_set(i) = point(2);
        heading_set(i) = proj_heading + atan(dl_set(i)/(1 - proj_kappa * l_set(i)));
        % 近似认为 kappa' == 0,frenet转cartesian公式，见第一章第三节评论区的链接
        kappa_set(i) = ((ddl_set(i) + proj_kappa * dl_set(i) * tan(heading_set(i) - proj_heading)) * ...
            (cos(heading_set(i) - proj_heading)^2)/(1 - proj_kappa * l_set(i)) + proj_kappa) * ...
            cos(heading_set(i) - proj_heading)/(1 - proj_kappa * l_set(i));
         
    end

end


function [proj_x,proj_y,proj_heading,proj_kappa] = CalcProjPoint(s,frenet_path_x,frenet_path_y,frenet_path_heading,...
    frenet_path_kappa,index2s)
% 该函数将计算在frenet坐标系下，点(s,l)在frenet坐标轴的投影的直角坐标(proj_x,proj_y,proj_heading,proj_kappa)'
% 先找匹配点的编号
    match_index = 1;
    while index2s(match_index) < s
        match_index = match_index + 1;
    end
    match_point = [frenet_path_x(match_index);frenet_path_y(match_index)];
    match_point_heading = frenet_path_heading(match_index);
    match_point_kappa = frenet_path_kappa(match_index);
    ds = s - index2s(match_index);
    match_tor = [cos(match_point_heading);sin(match_point_heading)];
    proj_point = match_point + ds * match_tor;
    proj_heading = match_point_heading + ds * match_point_kappa;
    proj_kappa = match_point_kappa;
    proj_x = proj_point(1);
    proj_y = proj_point(2);   
end

== matlab function testEmplanner_cs/Audi_A8_Sedan_1/decision&planning module/EM Planner2/calc path length and map between point and s ==
  data: trajectory_x input; path_s_end output; trajectory_y input; path_s output
function [path_s_end,path_s] = fcn(trajectory_x,trajectory_y)
% 该函数将计算以trajectory的s 与 x y 的对应关系，可以看作是trajectory index2s
n = length(trajectory_x);
path_s = zeros(n,1);
sum = 0;
for i = 2:length(trajectory_x)
    if isnan(trajectory_x(i))
        break;
    end
    sum = sum + sqrt((trajectory_x(i) - trajectory_x(i-1))^2 + (trajectory_y(i) - trajectory_y(i-1))^2);
    path_s(i) = sum;
end
% 计算出trajectory的长度
if i == n
    path_s_end = path_s(end);
else
    % 因为循环的退出条件为isnan(trajectory_x(i)) 所以 i 所对应的数为 nan 
    path_s_end = path_s(i - 1);
end

== matlab function testEmplanner_cs/Audi_A8_Sedan_1/decision&planning module/EM Planner2/calc plan start info and stitch trajectory ==
  data: pre_trajectory_x input; plan_start_x output; pre_trajectory_y input; pre_trajectory_heading input; pre_trajectory_kappa input; pre_trajectory_velocity input; pre_trajectory_accel input; pre_trajectory_time input; current_time input; host_x input; host_y input; host_heading_xy input; host_vx input; host_vy input; host_ax input; host_ay input; plan_start_y output; plan_start_heading output; plan_start_kappa output; plan_start_vx output; plan_start_vy output; plan_start_ax output; plan_start_ay output; plan_start_time output; stitch_x output; stitch_y output; stitch_heading output; stitch_kappa output; stitch_speed output; stitch_accel output; stitch_time output
function [plan_start_x,plan_start_y,plan_start_heading,plan_start_kappa,plan_start_vx,plan_start_vy,plan_start_ax,...
    plan_start_ay,plan_start_time,stitch_x,stitch_y,stitch_heading,stitch_kappa,stitch_speed,stitch_accel,stitch_time] ...
    = fcn(pre_trajectory_x,pre_trajectory_y,pre_trajectory_heading,pre_trajectory_kappa,pre_trajectory_velocity,...
    pre_trajectory_accel,pre_trajectory_time,current_time,host_x,host_y,host_heading_xy,host_vx,host_vy,host_ax,host_ay)
%该函数将计算规划的起点以及拼接轨迹的信息
%输入 上一周期的规划结果信息pre_trajectory x ,y,heading,kappa,velocity,accel,time
%     本周期的绝对时间current_time
%     定位信息host x,y,heading,kappa,vx,vy,ax,ay
%输出 规划起点信息plan_start x,y,heading,kappa,vx,vy,ax,ay(vx,vy,ax,ay)是世界坐标系的
%     待拼接的轨迹信息，一般在上一周期的轨迹中的current_time+100ms，往前取20个点。
%     当规划完成后，本周期的规划结果和stitch_trajectory一起拼好发给控制

%输出初始化
stitch_x = zeros(20,1);
stitch_y = zeros(20,1);
stitch_heading = zeros(20,1);
stitch_kappa = zeros(20,1);
stitch_speed = zeros(20,1);
stitch_accel = zeros(20,1);
%时间为负代表没有对应的拼接轨迹
stitch_time = ones(20,1)*-1;

%申明全局变量
persistent is_first_run;
if isempty(is_first_run)
    %代表代码首次运行
    is_first_run = 0;
    %按照轨迹拼接算法，应该用车辆动力学递推，但是首次运行车辆的速度都是0，所以没必要递推了
    plan_start_x = host_x;
    plan_start_y = host_y;
    plan_start_heading = host_heading_xy;
    plan_start_kappa = 0;
    plan_start_vx = 0;
    plan_start_vy = 0;
    plan_start_ax = 0;
    plan_start_ay = 0;
    %规划的起点的时间应该是当前时间+100ms
    plan_start_time = current_time + 0.1;
else
    %该函数不是首次运行
    x_cur = host_x;
    y_cur = host_y;
    heading_cur = host_heading_xy;
    kappa_cur = 0;
    %vx vy ax ay要转换成世界坐标系
    vx_cur = host_vx*cos(heading_cur) - host_vy*sin(heading_cur);
    vy_cur = host_vx*sin(heading_cur) + host_vy*cos(heading_cur);
    ax_cur = host_ax*cos(heading_cur) - host_ay*sin(heading_cur);
    ay_cur = host_ax*sin(heading_cur) + host_ay*cos(heading_cur);
    %规划周期
    dt = 0.1;
    %由于不是首次运行了，有上一时刻的轨迹了，找到上一周期轨迹规划的本周期车辆应该在的位置
    for i = 1:length(pre_trajectory_time) - 1
        if (pre_trajectory_time(i) <= current_time && pre_trajectory_time(i + 1) > current_time)
            break;
        end
    end
    %上一周期规划的本周期的车应该在的位置
    pre_x_desire = pre_trajectory_x(i);
    pre_y_desire = pre_trajectory_y(i);
    pre_heading_desire = pre_trajectory_heading(i);
    %计算横纵向误差
    %切向量
    tor = [cos(pre_heading_desire);sin(pre_heading_desire)];
    %法向量
    nor = [-sin(pre_heading_desire);cos(pre_heading_desire)];
    %误差向量
    d_err = [host_x;host_y] - [pre_x_desire;pre_y_desire];
    %纵向误差
    lon_err = abs(d_err'*tor);
    %横向误差
    lat_err = abs(d_err'*nor);
    %纵向误差大于2.5 横向误差大于0.5 认为控制没跟上
    if (lon_err > 2.5)||(lat_err > 0.5)
        %此分支处理控制未跟上的情况，规划起点通过运动学递推
        plan_start_x = x_cur + vx_cur * dt + 0.5 * ax_cur * dt * dt;
        plan_start_y = y_cur + vy_cur * dt + 0.5 * ay_cur * dt * dt;
        plan_start_vx = vx_cur + ax_cur * dt;
        plan_start_vy = vy_cur + ay_cur * dt;
        plan_start_heading = atan2(plan_start_vy,plan_start_vx);
        plan_start_ax = ax_cur;
        plan_start_ay = ay_cur;
        plan_start_kappa = kappa_cur;
        plan_start_time = current_time + 0.1;
        return;
    else
        %此分支表示控制能跟的上规划，开始拼接
        for j = i:length(pre_trajectory_time) - 1
            if (pre_trajectory_time(j) <= current_time + 0.1)&&(pre_trajectory_time(j + 1) > current_time + 0.1)
                break;
            end
        end
        %注：此算法要能运行需要trajectory的点有很高的密度
        plan_start_x = pre_trajectory_x(j);
        plan_start_y = pre_trajectory_y(j);
        plan_start_heading = pre_trajectory_heading(j);
        plan_start_kappa = pre_trajectory_kappa(j);
        %这里的pre_trajectory的速度,加速度是指轨迹的切向速度，切向加速度
        plan_start_vx = pre_trajectory_velocity(j) * cos(plan_start_heading);
        plan_start_vy = pre_trajectory_velocity(j) * sin(plan_start_heading);
        %pre_trajectory的加速度是切向加速度，要想计算ax,ay还要计算法向加速度
        %计算轨迹在current_time + 100ms 这个点的切向量法向量
        tor = [cos(plan_start_heading);sin(plan_start_heading)];
        nor = [-sin(plan_start_heading);cos(plan_start_heading)];
        a_tor = pre_trajectory_accel(j) * tor;
        a_nor = pre_trajectory_velocity(j)^2 * plan_start_kappa * nor ;
        plan_start_ax = a_tor(1) + a_nor(1);
        plan_start_ay = a_tor(2) + a_nor(2);
        plan_start_time = pre_trajectory_time(j);
        %计算拼接轨迹
        %j 表示 current_time + 0.1 的时间点在 pre_trajectory_time的编号
        %拼接是往从j开始，往前拼接20个，也就是pre_trajectory(j-1),j-2,j-3,....j-19
        %分两种情况，如果j小于20，意味着前面的轨迹点不够20个
        %如果j >= 20,意味着前面的点多于20个
        %还有一个细节需要考虑，pre_trajectory x(j) y(j) ....是规划的起点，那么在轨迹拼接时
        %需不需要在stitch_trajectory中把pre_trajectory x(j) y(j) ....包含进去
        %答案是否定的，不应该包进去，因为规划的起点会在规划模块计算完成后的结果中包含，如果在拼接的时候
        %还要包含，那就等于规划起点包含了两次
        %除非本周期计算的轨迹不包含规划起点，那么stitch_trajectory可以包含规划起点。
        %如果本周期计算的轨迹包含规划起点，那么stitch_trajectory就不可以包含规划起点。
        %我们选择规划包含起点，拼接不包含起点的做法
        
        %把起点去掉
        j = j - 1;
        if j >= 20
            stitch_x = pre_trajectory_x(j - 19:j);
            stitch_y = pre_trajectory_y(j - 19:j);
            stitch_heading = pre_trajectory_heading(j - 19:j);
            stitch_kappa = pre_trajectory_kappa(j - 19:j);
            stitch_speed = pre_trajectory_velocity(j - 19:j);
            stitch_accel = pre_trajectory_accel(j - 19:j);
            stitch_time = pre_trajectory_time(j - 19:j);
        else
            stitch_x(20 - j + 1:20) = pre_trajectory_x(1:j);
            stitch_y(20 - j + 1:20) = pre_trajectory_y(1:j);
            stitch_heading(20 - j + 1:20) = pre_trajectory_heading(1:j);
            stitch_kappa(20 - j + 1:20) = pre_trajectory_kappa(1:j);
            stitch_speed(20 - j + 1:20) = pre_trajectory_velocity(1:j);
            stitch_accel(20 - j + 1:20) = pre_trajectory_accel(1:j);
            stitch_time(20 - j + 1:20) = pre_trajectory_time(1:j);           
        end   
    end    
end

== matlab function testEmplanner_cs/Audi_A8_Sedan_1/decision&planning module/EM Planner2/genrate index to s ==
  data: path_x input; index2s output; path_y input; origin_x input; origin_y input; origin_match_point_index input
function index2s  = fcn(path_x,path_y,origin_x,origin_y,origin_match_point_index)
%该函数将输出index与s的转换关系，index2s表示当path_x,path_y的离散点的编号为i时，对应的弧长为index2s(i)
%输入 path_x path_y 待转化的离散点的集合
%     origin_x,y frenet原点在世界坐标系下的坐标
%     origin_match_point_index 原点的匹配点的编号
% path点的个数
n = 181;
% 输出初始化
index2s = zeros(n,1);
% 首先计算以path起点为坐标原点的index2s
for i = 2:n
    index2s(i) = sqrt((path_x(i) - path_x(i-1))^2 + (path_y(i) - path_y(i-1))^2) + index2s(i-1);
end
% 再计算以轨迹起点到frenet_path的坐标原点的弧长，记为s0，再用index2s - s0 就是最终的结果
% 计算s0
% s_temp frenet原点的匹配点的弧长
s_temp = index2s(origin_match_point_index);
%判断原点在匹配点的前面还是后面
%两个向量match_point_to_origin 
%        match_point_to_match_point_next
vector_match_2_origin = [origin_x;origin_y] - [path_x(origin_match_point_index);path_y(origin_match_point_index)];
vector_match_2_match_next = [path_x(origin_match_point_index + 1);path_y(origin_match_point_index + 1)] - ...
                            [path_x(origin_match_point_index);path_y(origin_match_point_index)];
if vector_match_2_origin'*vector_match_2_match_next > 0
    %坐标原点在匹配点的前面
    s0 = s_temp + sqrt(vector_match_2_origin'*vector_match_2_origin);
else
    %坐标原点在匹配点的后面
    s0 = s_temp - sqrt(vector_match_2_origin'*vector_match_2_origin);
end

index2s = index2s - ones(n,1)*s0;

== matlab function testEmplanner_cs/Audi_A8_Sedan_1/decision&planning module/EM Planner1/Cartesian2Frenet/MATLAB Function ==
  data: x_set input; s_set output; y_set input; frenet_path_x input; frenet_path_y input; proj_x_set input; proj_y_set input; proj_heading_set input; proj_match_point_index_set input; index2s input; l_set output
function [s_set,l_set] = fcn(x_set,y_set,frenet_path_x,frenet_path_y,...
    proj_x_set,proj_y_set,proj_heading_set,proj_match_point_index_set,index2s)
    %该函数将计算世界坐标系下的x_set，y_set上的点在frenet_path下的坐标s l
    %输入 x_set,y_set 待坐标转换的点
    %     frenet_path_x,frenet_path_y   frenet坐标轴
    %     proj_x,y,heading,kappa,proj_match_point_index 待坐标转换的点的投影点的信息
    %     index2s   frenet_path的index与s的转换表

    % 由于不知道有多少个点需要做坐标转换，所以需要做缓冲
    n = 128;%最多处理128个点
    %输出初始化
    s_set = ones(n,1)*nan;
    l_set = ones(n,1)*nan;
    for i = 1:length(x_set)
        if isnan(x_set(i))
            break;
        end
        %计算s，写个子函数
        s_set(i) = CalcSFromIndex2S(index2s,frenet_path_x,frenet_path_y,proj_x_set(i),proj_y_set(i),...
            proj_match_point_index_set(i));
        n_r = [-sin(proj_heading_set(i));cos(proj_heading_set(i))];
        r_h = [x_set(i);y_set(i)];
        r_r = [proj_x_set(i);proj_y_set(i)];
        l_set(i) = (r_h - r_r)'*n_r;
    end
end

function s = CalcSFromIndex2S(index2s,path_x,path_y,proj_x,proj_y,proj_match_point_index)
  %该函数将计算当指定index2s的映射关系后，计算点proj_x,proj_y的弧长
  vector_1 = [proj_x;proj_y] - [path_x(proj_match_point_index);path_y(proj_match_point_index)];
  %这里要考虑的更全面一些，因为要考虑到proj_match_point_index有可能在path的起点或终点
  if (proj_match_point_index < length(path_x))
      vector_2 = [path_x(proj_match_point_index + 1);path_y(proj_match_point_index + 1)] - ...
          [path_x(proj_match_point_index);path_y(proj_match_point_index)];
  else
      vector_2 = [path_x(proj_match_point_index);path_y(proj_match_point_index)] - ...
          [path_x(proj_match_point_index - 1);path_y(proj_match_point_index - 1)];
  end
  
  if vector_1'*vector_2 > 0
      s = index2s(proj_match_point_index) + sqrt(vector_1'*vector_1);
  else
      s = index2s(proj_match_point_index) - sqrt(vector_1'*vector_1);
  end
  
  
end
